simulink model "Lab4_DataLog_hw_solution"  (R2025b)
settings: Solver=FixedStepDiscrete  StartTime=0.0  StopTime=30  FixedStep=50e-6  RelTol=1e-3  EnableMultiTasking=on
undefined symbols (not defined in the file or in its folder): A0, A4, ADC, B0, C10, C11, C12, C13, C14, C15, C2, C3, C4, C5, CND4max, D0, D1, D10, D12, D13, D14, D2, D3, D4, D5, D6, D9, DiscIntNeverNeededParam, Max, MaxPer, ms, NumBits1, NumBits2, P1, P17, P20, P35, P36, P37, P38, P43, P44, P45, P46, P47, P48, P49, P50, P51, P52, P54, P55, P58, P59, P61, P62, P63, Pin, PWM1_Trg1, Resol ... (+2)
libraries: simulink x31, MCHP_Blockset x20
(part 3 of 5)

== system Lab4_DataLog_hw_solution/Bipolar to Unipolar PWM input set for input in [0 1] ==
  note: Output default value is 0.5 on all 3 channels enabling current bias estimator
  In [-1 1] : Inport
  Enable : EnablePort
  Bias : Bias  Bias=0.5  SaturateOnIntegerOverflow=off
  Gain : Gain  Gain=0.5
  Out [0 1] : Outport  OutputWhenDisabled=reset  InitialOutput=[0.5 0.5 0.5]'
  wires:
  Bias/1 -> Out [0 1]/1
  Gain/1 -> Bias/1
  In [-1 1]/1 -> Gain/1

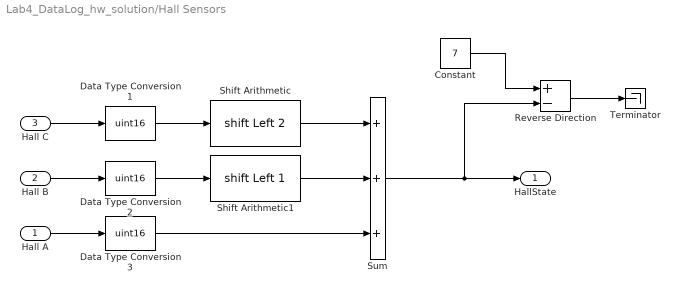
== system Lab4_DataLog_hw_solution/Hall Sensors ==
  Hall A : Inport
  Hall B : Inport  Port=2
  Hall C : Inport  Port=3
  Constant : Constant  Value=7  OutDataTypeStr=uint16
  Data Type Conversion1 : DataTypeConversion  OutDataTypeStr=uint16  RndMeth=Simplest  SaturateOnIntegerOverflow=off
  Data Type Conversion2 : DataTypeConversion  OutDataTypeStr=uint16  RndMeth=Simplest  SaturateOnIntegerOverflow=off
  Data Type Conversion3 : DataTypeConversion  OutDataTypeStr=uint16  RndMeth=Simplest  SaturateOnIntegerOverflow=off
  Reverse Direction : Sum  Inputs=+-
  Shift Arithmetic : ArithShift  BitShiftNumber=2  BitShiftDirection=Left
  Shift Arithmetic1 : ArithShift  BitShiftNumber=1  BitShiftDirection=Left
  Sum : Sum  Inputs=+++
  Terminator : Terminator
  HallState : Outport
  wires:
  Data Type Conversion2/1 -> Shift Arithmetic1/1
  Data Type Conversion3/1 -> Sum/3
  Data Type Conversion1/1 -> Shift Arithmetic/1
  Shift Arithmetic1/1 -> Sum/2
  Shift Arithmetic/1 -> Sum/1
  Sum/1 -> Reverse Direction/2, HallState/1
  Hall B/1 -> Data Type Conversion2/1
  Hall C/1 -> Data Type Conversion1/1
  Hall A/1 -> Data Type Conversion3/1
  Constant/1 -> Reverse Direction/1
  Reverse Direction/1 -> Terminator/1

== system Lab4_DataLog_hw_solution/R(theta) rotation builder ==
  note: $\textbf{Rotation matrix builder}\\\text{Builds } R(\theta) \text{ from the rotor electrical angle } \theta.\\R(\theta) \text{ is used for inverse Park } (dq \rightarrow \alpha\beta);\\R(\theta)^{T} \text{ is used for Park } (\alpha\beta \rightarrow dq).$
  theta : Inport
  Mux : Mux  Inputs=2
  Rot : Subsystem
  Sin : Trigonometry  Operator=sincos
  R : Outport
  wires:
  Rot/1("Rot ") -> R/1
  Sin/2 -> Mux/2
  theta/1 -> Sin/1
  Sin/1 -> Mux/1
  Mux/1 -> Rot/1(sin cos)

== system Lab4_DataLog_hw_solution/SineWave Generator ==
  note: $\textbf{Angle generator}\\\text{The uint32 integrator wraps by natural overflow (modulo } 2^{32} \text{).}\\\text{For the integer code } k = 0 \ldots 2^{32}, \text{ the output gain gives}\\\theta = \frac{2\pi\,k}{2^{32}} \in [0,\,2\pi[\quad\text{(} 0 \text{ and } 2\pi \text{ are the same angle).}$
  Freq (Hz) : Inport  Unit=Hz  PortDimensions=1
  Angle PU 0 2^32 : DiscreteIntegrator  gainval=(2^32)  SampleTime=50e-6  OutDataTypeStr=uint32  ICPrevOutput=DiscIntNeverNeededParam  ICPrevScaledInput=DiscIntNeverNeededParam
  Angle radian : Gain  Gain=2*pi/2^32  OutDataTypeStr=single
  Angle : Outport
  wires:
  Angle PU 0 2^32/1 -> Angle radian/1
  Freq (Hz)/1 -> Angle PU 0 2^32/1
  Angle radian/1 -> Angle/1

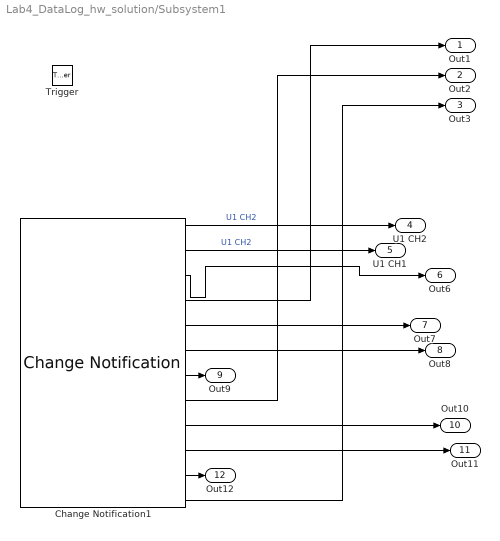
== system Lab4_DataLog_hw_solution/Subsystem1 ==
  Trigger : TriggerPort  TriggerType=function-call  VariantControl=(inherit)  PortDimensions=1
  Change Notification1 : MCHP_Blockset/Pulse Input//Output/Change Notification  IntPriority=5  Channel="[19    20    21]"  Channel_EP="[  D4  D5  D6]"  Channel_OLD="[52  53  54]"  Channel_UP_Down_Periode="[3     3     3]"  MaxChannel="[1     1     1]"  SafeMarge="[0     0     0]"  MaxChannelValue="2.^[ 27.575  27.575  27.575]  =>  [199999999  199999999  199999999]"  CNxmax="[199999999  199999999  199999999]"  Timer="[4  4  4]"  ChangeDetected="[3     3     3]"  OutputPortValue="[1     1     1]"  TimerBitWidth=32 bits  TimerBitWidth_fixed=16 bits  evalin_ws=CND4max=MCHP_Fun.Hex2num('41A7D783FE000000');CND5max=MCHP_Fun.Hex2num('41A7D783FE000000');CND6max=MCHP_Fun.Hex2num('41A7D783FE000000');  SampleTime=-1  Status=OK  MCHP_USER_INTERRUPTS={CNDIE}{CND}{Change Notification - D}{5};  MCHP_PORT={Change Notification D4}{CND4}9:0:D4;{Change Notification D5}{CND5}9:0:D5;{Change Notification D6}{CND6}9:0:D6;  MCHP_TIMER_REQUEST="{Change Notification 52}{CND4}7:33:1:0:[4   5   6   7   8   9  10  11  12]:100000000;{Change Notification 53}{CND5}7:33:1:0:[4   5   6   7   8   9  10  11  12]:100000000;{Change Notification 54}{CND6}7:33:1:0:[4   5   6   7   8   9  10  11  12]:100000000;"  MCHP_TIMER_RESULT=[4 199999998.99999982119 32 ;4 199999998.99999982119 32 ;4 199999998.99999982119 32 ]  MCHP_MASTERLINK=Lab4_DataLog_hw_solution/BOARD MCLV-48V-300W dsPIC33AK512MC510 MC DIM1/Microchip Master
      settings: SourceProductName=MPLAB Device Blocks for Simulink
  Out1 : Outport
  Out2 : Outport  Port=2
  Out3 : Outport  Port=3
  U1 CH2 : Outport  Port=4
  U1 CH1 : Outport  Port=5
  Out6 : Outport  Port=6
  Out7 : Outport  Port=7
  Out8 : Outport  Port=8
  Out9 : Outport  Port=9
  Out10 : Outport  Port=10
  Out11 : Outport  Port=11
  Out12 : Outport  Port=12
  wires:
  Change Notification1/12 -> Out3/1
  Change Notification1/9 -> Out10/1
  Change Notification1/8 -> Out2/1
  Change Notification1/1 -> U1 CH2/1  "U1 CH2"
  Change Notification1/6 -> Out8/1
  Change Notification1/3 -> Out6/1
  Change Notification1/10 -> Out11/1
  Change Notification1/2 -> U1 CH1/1  "U1 CH2"
  Change Notification1/5 -> Out7/1
  Change Notification1/4 -> Out1/1
  Change Notification1/7 -> Out9/1
  Change Notification1/11 -> Out12/1

== system Lab4_DataLog_hw_solution/dq to abc (Inverse Park + Inverse Clarke) ==
  note: $\textbf{Inverse Clarke}\;(\alpha\beta \rightarrow abc)\\a = \alpha\\b = -\frac{1}{2}\alpha + \frac{\sqrt{3}}{2}\beta\\c = -\frac{1}{2}\alpha - \frac{\sqrt{3}}{2}\beta\\\text{zero-sequence-free inverse } (a+b+c=0)$
  dq : Inport
  R : Inport  Port=2
  Data Type Duplicate : DataTypeDuplicate
  Inverse Clarke : Gain  Gain=|  Multiplication=Matrix(K*u)  RndMeth=Round  OutDataTypeStr=Inherit: Same as input
      | [1   -1/2        -1/2;
      |         0   sqrt(3)/2   -sqrt(3)/2]'
  Inverse Park : Product  Multiplication=Matrix(*)  OutDataTypeStr=Inherit: Inherit via back propagation  RndMeth=Round
  abc : Outport
  wires:
  Inverse Clarke/1 -> abc/1
  Inverse Park/1 -> Inverse Clarke/1, Data Type Duplicate/1
  dq/1 -> Inverse Park/2, Data Type Duplicate/2
  R/1 -> Inverse Park/1
